simulink model "Sample_Project_s32k144"  (R2019a)
settings: Solver=FixedStepDiscrete  StartTime=0.0  StopTime=10  FixedStep=0.01  RelTol=1e-3
InitFcn:
  | mbd_s32k_consistency_checks(bdroot(gcs));
undefined symbols (not defined in the file): LQFP
libraries: mbd_s32k1xx_ec_toolbox x19, canmsglib x3, simulink x1
Description:
  | This model demonstrate the "GPIO" block functionality.
  | 
  | Validation:
  | - Blue LED is blinking during execution
  | - Press SW2 to light a Green LED
settings Model: Creator=NXP MBDT Team  LastModifiedBy=marsh
settings DataIOCC: ExternalInput=off  InitialState=off  LimitDataPoints=on  SaveFormat=Array  SaveOutput=off  SignalLogging=off  SaveTime=off  ReturnWorkspaceOutputs=off
settings OptimizationCC: DefaultParameterBehavior=Inlined  UseDivisionForNetSlopeComputation=on  GainParamInheritBuiltInType=on  UseFloatMulNetSlope=on  InlineInvariantSignals=on  EnhancedBackFolding=on  PassReuseOutputArgsAs=Individual arguments  ZeroExternalMemoryAtStartup=off  ZeroInternalMemoryAtStartup=off  NoFixptDivByZeroProtection=on  EfficientFloat2IntCast=on  OptimizeBlockOrder=speed  DifferentSizesBufferReuse=on  OptimizationCustomize=off
settings DebuggingCC: UnderspecifiedInitializationDetection=Classic  MergeDetectMultiDrivingBlocksExec=none  SolverPrmCheckMsg=warning  InheritedTsInSrcMsg=none  SingleTaskRateTransMsg=error  ParameterTunabilityLossMsg=error  UnconnectedInputMsg=error  UnconnectedOutputMsg=error  UnconnectedLineMsg=error  AllowSymbolicDim=off  UnknownTsInhSupMsg=error  StateNameClashWarn=warning  SFUnexpectedBacktrackingDiag=warning  SFNoUnconditionalDefaultTransitionDiag=warning  SFExecutionAtInitializationDiag=none  ArithmeticOperatorsInVariantConditions=warning
settings HardwareCC: ProdBitPerPointer=32  ProdBitPerSizeT=32  ProdBitPerPtrDiffT=32  ProdLargestAtomicInteger=Long  ProdLargestAtomicFloat=Double  ProdWordSize=32  ProdLongLongMode=on  ProdHWDeviceType=ARM Compatible->ARM Cortex
settings ModelReferenceCC: PropagateSignalLabelsOutOfModel=off
settings SFSimCC: SimUseLocalCustomCode=off  MATLABDynamicMemAlloc=off
settings RTWCC: SystemTargetFile=mbd_s32k.tlc  MakeCommand=mbd_s32k_make_rtw COPY_MDLREF_INCLUDES=0  TemplateMakefile=mbd_s32k.tmf  Description=Model Based Design Toolbox S32K1xx Code Generation Target  GenerateReport=on  RTWUseLocalCustomCode=off  IncludeHyperlinkInReport=on  LaunchReport=on  GenerateTraceInfo=on  GenerateTraceReport=on  GenerateTraceReportSl=on  GenerateTraceReportSf=on  GenerateTraceReportEml=on  GenerateCodeMetricsReport=on
settings CodeAppCC: ForceParamTrailComments=on  IgnoreCustomStorageClasses=off  OperatorAnnotations=on  SimulinkDataObjDesc=on  SFDataObjDesc=on  CustomSymbolStrGlobalVar=rt$N$M  CustomSymbolStrType=$N$M  CustomSymbolStrFcn=$N$M$F  CustomSymbolStrMacro=$N$M  InsertBlockDesc=on
settings STFCustomTargetCC: TargetLangStandard=C99 (ISO)  MultiwordLength=256  ModelReferenceCompliant=off  CombineOutputUpdateFcns=on  ERTCustomFileBanners=on  SupportContinuousTime=off  SupportNonInlinedSFcns=off  RemoveResetFunc=on  MATLABClassNameForMDSCustomization=Simulink.SoftwareTarget.ERTCustomization  GRTInterface=off  SystemTargetFile=mbd_s32k.tlc
settings ERTTargetCC: TargetLangStandard=C99 (ISO)  ModelReferenceCompliant=off  ParMdlRefBuildCompliant=off  CompOptLevelCompliant=off  ConcurrentExecutionCompliant=off  ModelStepFunctionPrototypeControlCompliant=off  CPPClassGenCompliant=off  UseToolchainInfoCompliant=off  InlinedParameterPlacement=NonHierarchical  ERTCustomFileTemplate=example_file_process.tlc
settings ConfigComp: CovMetricSettings=dw  CovHtmlReporting=on  CovSaveCumulativeToWorkspaceVar=on  CovSaveSingleToWorkspaceVar=on  CovExternalEMLEnable=off

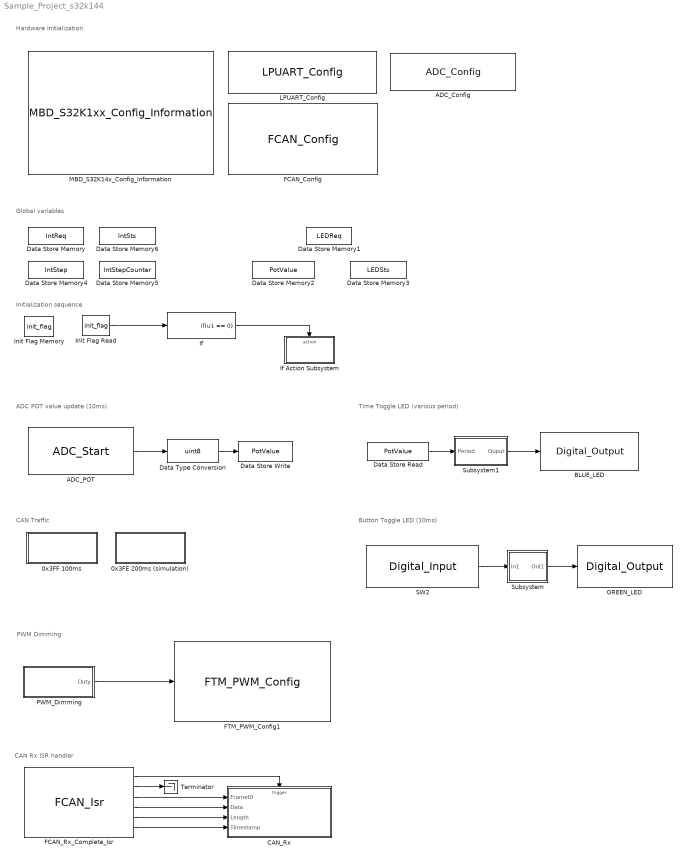
== system Sample_Project_s32k144 ==
  note: ADC POT value update (10ms)
  note: CAN Rx ISR handler
  note: CAN Traffic
  note: Button Toggle LED (10ms)
  note: Time Toggle LED (various period)
  note: Hardware Initialization
  note: Global variables
  note: Initialization sequence
  note: PWM Dimming
  0x3FE 200ms (simulation) : Subsystem
  0x3FF 100ms : Subsystem
  ADC_Config : mbd_s32k1xx_ec_toolbox/Motor Control Blocks/ADC Blocks/ADC_Config  Priority=1  instance=0  mode=8-bit conversion  smplts=29  adiclk=alternate clock 1  adiv=input clock  show_adv_opts=on  pretrgsel=Software pre-trigger  swpretrg=Disabled  adtrg=software  trgsel=PDB output  refsel=Vrefh and Vrefl  supply_monitoring=off  acfe=off  acfgt=off  acren=off  cv1=0  cv2=0  adco=off  avge=off  avgs=4 samples
  ADC_POT : mbd_s32k1xx_ec_toolbox/Motor Control Blocks/ADC Blocks/ADC_Start  Priority=2  instance=0  adc_r=A  adc_chan=PTC14: [ADC0_SE12 | ADC Single Ended Input]  aien=off  mcuTargetUpdate=on
  BLUE_LED : mbd_s32k1xx_ec_toolbox/GPIO Blocks/Digital_Output  gpio_pin=PTD0: [PTD0 | Port D I/O]  init_val=Low  drive_strength=Low
  CAN_Rx : Subsystem  TreatAsAtomicUnit=on
      settings: RTWSystemCode=Nonreusable function
  Data Store Memory : DataStoreMemory  DataStoreName=IntReq  ReadBeforeWriteMsg=warning  WriteAfterWriteMsg=warning  WriteAfterReadMsg=warning  ShowAdditionalParam=off  OutDataTypeStr=uint8
  Data Store Memory1 : DataStoreMemory  DataStoreName=LEDReq  ReadBeforeWriteMsg=warning  WriteAfterWriteMsg=warning  WriteAfterReadMsg=warning  ShowAdditionalParam=off  OutDataTypeStr=boolean
  Data Store Memory2 : DataStoreMemory  DataStoreName=PotValue  ReadBeforeWriteMsg=warning  WriteAfterWriteMsg=warning  WriteAfterReadMsg=warning  InitialValue=0.1  ShowAdditionalParam=off  OutMin=[0.1]  OutMax=[2.65]  OutDataTypeStr=uint8
  Data Store Memory3 : DataStoreMemory  DataStoreName=LEDSts  ReadBeforeWriteMsg=warning  WriteAfterWriteMsg=warning  WriteAfterReadMsg=warning  ShowAdditionalParam=off  OutDataTypeStr=boolean
  Data Store Memory4 : DataStoreMemory  DataStoreName=IntStep  ReadBeforeWriteMsg=warning  WriteAfterWriteMsg=warning  WriteAfterReadMsg=warning  ShowAdditionalParam=off  OutDataTypeStr=double
  Data Store Memory5 : DataStoreMemory  DataStoreName=IntStepCounter  ReadBeforeWriteMsg=warning  WriteAfterWriteMsg=warning  WriteAfterReadMsg=warning  ShowAdditionalParam=off  OutDataTypeStr=uint8
  Data Store Memory6 : DataStoreMemory  DataStoreName=IntSts  ReadBeforeWriteMsg=warning  WriteAfterWriteMsg=warning  WriteAfterReadMsg=warning  ShowAdditionalParam=off  OutDataTypeStr=double
  Data Store Read : DataStoreRead  DataStoreName=PotValue
  Data Store Write : DataStoreWrite  DataStoreName=PotValue
  Data Type Conversion : DataTypeConversion  OutDataTypeStr=uint8
  FCAN_Config : mbd_s32k1xx_ec_toolbox/Communication Blocks/CAN Blocks/FCAN_Config  Priority=1  can_instance=0  can_mode=Loop-back mode  can_max_num_mb=16  can_rx=PTE4: [CAN0_RX | CAN Rx channel]  can_tx=PTE5: [CAN0_TX | CAN Tx Channel]  show_adv_opts=on  can_clk_src=Peripheral clock  bitrate=500  bitrate_adv_opts=off  can_presdiv=7  can_rjw=3  can_pseg1=6  can_pseg2=3  can_propseg=7  can_cbt_presdiv=9  can_cbt_rjw=0  can_cbt_pseg1=3  can_cbt_pseg2=3  can_cbt_propseg=6  can_fd_enable=off  can_payload=8  can_rxfifo_enable=off  can_fifo_id_filter_extended=off  can_fifo_id_filter_remote=off  can_num_id_filters=8  can_fifo_id_format=A  can_fifo_id_filter={'0x0', '0x0', '0x0', '0x0', '0x0', '0x0', '0x0', '0x0'}  can_pn_enable=off  can_wakeup_match=off  can_wakeup_timeout=off  can_timeout_en=off  can_match_timeout=1  can_multiple_matches_en=off  can_num_matches=1  can_idfilter_extendedid=off  can_idfilter_remoteframe=off  can_idfilter_type=Match exact  can_idfilter_id1=0  can_idfilter_id2=0  can_payloadfilter_enable=on  can_payloadfilter_dlclow=0  can_payloadfilter_dlchigh=0  can_payloadfilter_type=Match exact  can_payloadfilter_payload1_b0=0  can_payloadfilter_payload1_b1=0  can_payloadfilter_payload1_b2=0  can_payloadfilter_payload1_b3=0  can_payloadfilter_payload1_b4=0  can_payloadfilter_payload1_b5=0  can_payloadfilter_payload1_b6=0  can_payloadfilter_payload1_b7=0  can_payloadfilter_payload2_b0=0  can_payloadfilter_payload2_b1=0  can_payloadfilter_payload2_b2=0  can_payloadfilter_payload2_b3=0  can_payloadfilter_payload2_b4=0  can_payloadfilter_payload2_b5=0  can_payloadfilter_payload2_b6=0  can_payloadfilter_payload2_b7=0
  FCAN_Rx_Complete_Isr : mbd_s32k1xx_ec_toolbox/Communication Blocks/CAN Blocks/FCAN_Isr  can_instance=0  can_event=Rx Complete
  FTM_PWM_Config1 : mbd_s32k1xx_ec_toolbox/Motor Control Blocks/FTM Blocks/FTM_PWM_Config  Priority=1  ftmModule=0  ftmMode=Edge-Aligned PWM  ftmSourceClock=80 MHz  swcontrol_enable=off  chan0En=on  chan0Type=Complementary  chan2En=off  chan2Type=Independent  chan4En=off  chan4Type=Independent  chan6En=off  chan6Type=Independent  ftmPwmUnits=Hz  outFrequency=5000  ftmPeriod=16000  ftmPrescaler=Divide by 1  deadtimeUnits=Nanoseconds  deadtimeNs=1000  deadtimeTicks=20  deadtimePrescaler=Divide by 4  dutyCycleCh0=0.5  dutyCycleCh1=0.1  dutyCycleCh2=0  dutyCycleCh3=0  dutyCycleCh4=0.25  dutyCycleCh5=0.25  dutyCycleCh6=0.25  dutyCycleCh7=0.25  dutyCycleSim=off  startAfterInit=on  showAdvOpt=on  pinFtmCh0=PTD15: [FTM0_CH0 | FTM Channel]  pinFtmCh1=None  pinPolCh0=Active High  pinPolCh1=Active Low  outputComplem0=Main duplicated  outputLevel0=Low  outputLevel1=Low  pinFtmCh2=PTB14: [FTM0_CH2 | FTM Channel]  pinFtmCh3=None  pinPolCh2=Active High  pinPolCh3=Active Low  outputComplem2=Main duplicated  outputLevel2=Low  outputLevel3=Low  pinFtmCh4=PTB4: [FTM0_CH4 | FTM Channel]  pinFtmCh5=None  pinPolCh4=Active High  pinPolCh5=Active Low  outputComplem4=Main duplicated  outputLevel4=Low  outputLevel5=Low  pinFtmCh6=PTA17: [FTM0_CH6 | FTM Channel]  pinFtmCh7=None  pinPolCh6=Active Low  pinPolCh7=Active Low  outputComplem6=Main duplicated  outputLevel6=Low  outputLevel7=Low  initTrigger=off  chTrigger0=on  chTrigger1=off  chTrigger2=off  chTrigger3=off  chTrigger4=off  chTrigger5=off  chTrigger6=off  chTrigger7=off  mcuTargetUpdate=on  pwmSyncTrg=Software trigger  pwmSyncHwRouting=TRGMUX_FTM7  pwmSyncTrg0=on  pwmSyncTrg1=on  pwmSyncTrg2=on  pwmSyncAutoClear=on  pwmSyncMinLoad=on  pwmSyncMaxLoad=on  pwmSyncInvert=System Clock  pwmSyncOutControl=System Clock  pwmSyncOutMask=System Clock  pwmSyncCounterInitial=System Clock  pwmSyncPoints=Update now  reloadEnable=off  reloadPriority=15  reloadHalfCycle=off  reloadHCR=0  reloadFrequency=0  chnMatch0=off  chnMatch1=off  chnMatch2=off  chnMatch3=off  chnMatch4=off  chnMatch5=off  chnMatch6=off  chnMatch7=off  pwmFaultProtection=off  pwmFaultInterrupt=off  pwmFaultClearing=Automatic Fault control for all channels  pwmFaultPinState=Safe Value  pwmFaultFilterValue=2  pwmFaultPriority=0  fault_disen_0=off  fault_filter_0=off  fault_polarity_0=Active Low  fault_disen_1=off  fault_filter_1=off  fault_polarity_1=Active high  fault_disen_2=off  fault_filter_2=off  fault_polarity_2=Active high  fault_disen_3=off  fault_filter_3=off  fault_polarity_3=Active high  fault_pin_0=None  fault_pin_1=None  fault_pin_2=None  fault_pin_3=None
  GREEN_LED : mbd_s32k1xx_ec_toolbox/GPIO Blocks/Digital_Output  gpio_pin=PTD16: [PTD16 | Port D I/O]  init_val=Low  drive_strength=Low
  If : If  IfExpression=u1 == 0  ShowElse=off
  If Action Subsystem : Subsystem  TreatAsAtomicUnit=on
  Init Flag Memory : DataStoreMemory  DataStoreName=init_flag  ReadBeforeWriteMsg=warning  WriteAfterWriteMsg=warning  WriteAfterReadMsg=warning  ShowAdditionalParam=off  OutDataTypeStr=uint32
  Init Flag Read : DataStoreRead  DataStoreName=init_flag
  LPUART_Config : mbd_s32k1xx_ec_toolbox/Communication Blocks/UART Blocks/LPUART_Config  Priority=1  instance=1  baudrate=115200  databits=8  parity=None  sbns=1  bothedge=rising edge  rxinv=off  txinv=off  show_adv_opts=on  brk13=13 - 16 bit times  lbkde=13 - 16 bit times  rx=PTC6: [LPUART1_RX | Receive]  tx=PTC7: [LPUART1_TX | Transmit]  cts=PTA6: [LPUART1_CTS | Clear To Send (bar)]  rts=PTA7: [LPUART1_RTS | Request To Send]
  MBD_S32K14x_Config_Information : mbd_s32k1xx_ec_toolbox/MBD_S32K1xx_Config_Information  mbdt_ver=0  disp_str=|  config_params=[]  mcu_target_name=S32K144  mcu_target_package=100-LQFP  mcu_target_sram_size=64KB  mcu_system_clock_freq=80  mcu_xtal_freq=External 8  mcu_steptick_timer=LPIT Channel 0  mcu_steptick_prio=15  ds_import_enable=on  target_compiler=GCC  target_memory=FLASH  gcc_target_compile_opts=-mcpu=cortex-m4 -mthumb -mfloat-abi=hard -mfpu=fpv4-sp-d16 -O1 -g -gstrict-dwarf  gcc_target_assemble_opts=-mcpu=cortex-m4 -mthumb -mfloat-abi=hard -mfpu=fpv4-sp-d16 -g  gcc_target_link_opts=-mcpu=cortex-m4 -mthumb -mfloat-abi=hard -mfpu=fpv4-sp-d16  gcc_target_default_lcf=on  gcc_target_user_lcf=S32K148_192_flash.ld  ghs_target_compile_opts=-cpu=cortexm4f -thumb -DARM_MATH_CM4 -fpu=vfpv4_d16 -fsingle -Ogeneral -Wundef -Wimplicit-int -Wshadow -Wtrigraphs --no_commons --gnu_asm -gnu99 -gdwarf-2 -G  ghs_target_assemble_opts=-cpu=cortexm4f -fpu=vfpv4_d16  ghs_target_link_opts=-cpu=cortexm4f -thumb -fpu=vfpv4_d16  ghs_target_default_lcf=on  ghs_target_user_lcf=S32K148_192_flash.ld  iar_target_compile_opts=--cpu=Cortex-M4F --thumb --fpu=VFPv4_sp -Ol -e --debug --dlib_config normal  iar_target_assemble_opts=--cpu Cortex-M4F --thumb --fpu VFPv4_sp  iar_target_link_opts=--no_exceptions --vfe --inline  iar_target_default_lcf=on  iar_target_user_lcf=S32K148_192_flash.icf  pil_download_enable=on  rbl_download_enable=on  rbl_start_delay=5000000  rbl_download_interface=OpenSDA  rbl_restart_request=off  rbl_com_port=COM5  rbl_com_port_custom=COM1  pil_download_rate=115200  pil_opensda_drive=E: EVB-S32K144  pil_opensda_drive_custom=D  pil_uart_instance=1  pil_uart_rx=PTC6: [LPUART1_RX | Receive]  pil_uart_tx=PTC7: [LPUART1_TX | Transmit]  FTM_PWM_PcrCheckEnDis=on  FTM_Input_Edge_Inputs_PcrCheckEnDis=on  FTM_Dual_Edge_Inputs_PcrCheckEnDis=on  FTM_Quadrature_Inputs_PcrCheckEnDis=on  FTM_Hall_Sensor_Inputs_PcrCheckEnDis=on  LPTMR_PcrCheckEnDis=on  PIT_PcrCheckEnDis=on  RTC_PcrCheckEnDis=on  FlexCAN_PcrCheckEnDis=on  LIN_PcrCheckEnDis=on  FlexIO_PcrCheckEnDis=on  LPI2C_PcrCheckEnDis=on  LPSPI_PcrCheckEnDis=on  LPUART_PcrCheckEnDis=on  CMP_PcrCheckEnDis=on  GPIO_OutputPcrCheckEnDis=on  GPIO_InputPcrCheckEnDis=on  SBC_PcrCheckEnDis=on  AMMCLIB_PcrCheckEnDis=on  FM_PcrCheckEnDis=on  Profile_PcrCheckEnDis=on  ConfigParams_PcrCheckEnDis=on  ModelRef_PcrCheckEnDis=on  PDB0_PcrCheckEnDis=on  CSEc_PcrCheckEnDis=on  eDMA_PcrCheckEnDis=on  ADC_PcrCheckEnDis=on  WDOG_PcrCheckEnDis=on
      | Target : S32K144-64KB_SRAM
      | Package : 100-pin
      | System clock : 80 MHz
      | XTAL clock : External 8 MHz
      | Compiler : IAR
      | Target Type : FLASH
      | Download Code after build : off
      | Step Tick Interrupt Priority : 15
  PWM_Dimming : Subsystem
  SW2 : mbd_s32k1xx_ec_toolbox/GPIO Blocks/Digital_Input  gpio_pin=PTC12: [PTC12 | Port C I/O]  pull_resistor=Pulldown  passive_filter=off
  Subsystem : Subsystem
  Subsystem1 : Subsystem
  Terminator : Terminator
  wires:
  SW2/1 -> Subsystem/1(In1)
  Subsystem/1(Out1) -> GREEN_LED/1
  Data Store Read/1 -> Subsystem1/1(Period)
  If/1 -> If Action Subsystem/Action
  Init Flag Read/1 -> If/1
  FCAN_Rx_Complete_Isr/2 -> Terminator/1
  FCAN_Rx_Complete_Isr/4 -> CAN_Rx/2("Data ")
  FCAN_Rx_Complete_Isr/5 -> CAN_Rx/3(Length)
  FCAN_Rx_Complete_Isr/1 -> CAN_Rx/Trigger
  FCAN_Rx_Complete_Isr/3 -> CAN_Rx/1(FrameID)
  FCAN_Rx_Complete_Isr/6 -> CAN_Rx/4(Timestamp)
  ADC_POT/1 -> Data Type Conversion/1
  Data Type Conversion/1 -> Data Store Write/1
  Subsystem1/1(Ouput) -> BLUE_LED/1
  PWM_Dimming/1(Duty) -> FTM_PWM_Config1/1

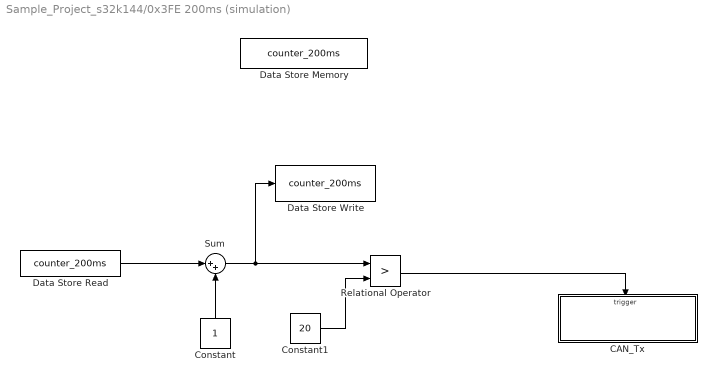
== system Sample_Project_s32k144/0x3FE 200ms (simulation) ==
  CAN_Tx : Subsystem  TreatAsAtomicUnit=on
      settings: RTWSystemCode=Nonreusable function
  Constant : Constant  OutDataTypeStr=uint8
  Constant1 : Constant  Value=20
  Data Store Memory : DataStoreMemory  DataStoreName=counter_200ms  ReadBeforeWriteMsg=warning  WriteAfterWriteMsg=warning  WriteAfterReadMsg=warning  ShowAdditionalParam=off  OutDataTypeStr=uint8
  Data Store Read : DataStoreRead  DataStoreName=counter_200ms
  Data Store Write : DataStoreWrite  DataStoreName=counter_200ms
  Relational Operator : RelationalOperator  Operator=>  OutDataTypeStr=boolean  RndMeth=Simplest
  Sum : Sum  Inputs=|++  AccumDataTypeStr=uint8
  wires:
  Constant1/1 -> Relational Operator/2
  Relational Operator/1 -> CAN_Tx/Trigger
  Constant/1 -> Sum/2
  Sum/1 -> Data Store Write/1, Relational Operator/1
  Data Store Read/1 -> Sum/1

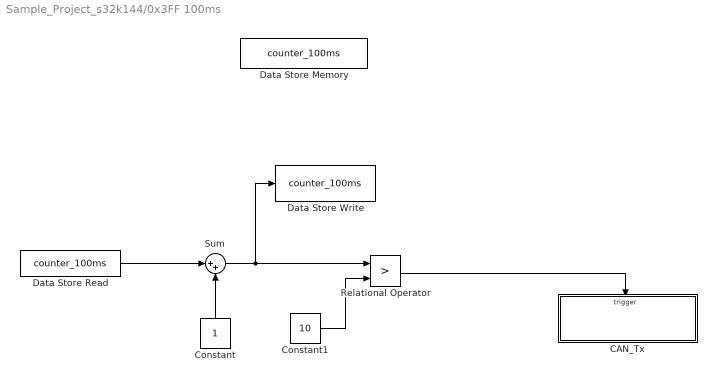
== system Sample_Project_s32k144/0x3FF 100ms ==
  CAN_Tx : Subsystem  TreatAsAtomicUnit=on
      settings: RTWSystemCode=Nonreusable function
  Constant : Constant  OutDataTypeStr=uint8
  Constant1 : Constant  Value=10
  Data Store Memory : DataStoreMemory  DataStoreName=counter_100ms  ReadBeforeWriteMsg=warning  WriteAfterWriteMsg=warning  WriteAfterReadMsg=warning  ShowAdditionalParam=off  OutDataTypeStr=uint8
  Data Store Read : DataStoreRead  DataStoreName=counter_100ms
  Data Store Write : DataStoreWrite  DataStoreName=counter_100ms
  Relational Operator : RelationalOperator  Operator=>  OutDataTypeStr=boolean  RndMeth=Simplest
  Sum : Sum  Inputs=|++  AccumDataTypeStr=uint8
  wires:
  Constant1/1 -> Relational Operator/2
  Relational Operator/1 -> CAN_Tx/Trigger
  Constant/1 -> Sum/2
  Sum/1 -> Data Store Write/1, Relational Operator/1
  Data Store Read/1 -> Sum/1

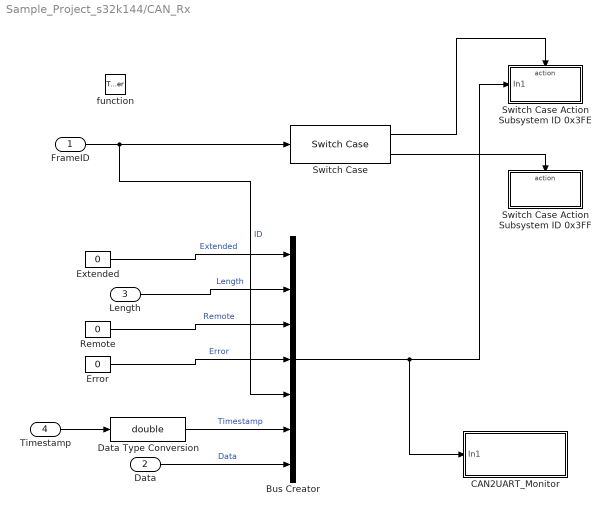
== system Sample_Project_s32k144/CAN_Rx ==
  FrameID : Inport
  "Data " : Inport  Port=2
  Length : Inport  Port=3
  Timestamp : Inport  Port=4
  function : TriggerPort  TriggerType=function-call  VariantControl=Variant
  Bus Creator : BusCreator  Inputs=7  OutDataTypeStr=Bus: CAN_MESSAGE_BUS  NonVirtualBus=on
  CAN2UART_Monitor : Subsystem
  Data Type Conversion : DataTypeConversion  OutDataTypeStr=double
  Error : Constant  Value=0  OutDataTypeStr=uint8
  Extended : Constant  Value=0  OutDataTypeStr=uint8
  Remote : Constant  Value=0  OutDataTypeStr=uint8
  Switch Case : SwitchCase  CaseConditions={hex2dec('3FE'), hex2dec('3FF')}  ShowDefaultCase=off
  Switch Case Action Subsystem ID 0x3FE : Subsystem  TreatAsAtomicUnit=on
  Switch Case Action Subsystem ID 0x3FF : Subsystem  TreatAsAtomicUnit=on
  wires:
  FrameID/1 -> Bus Creator/5, Switch Case/1  "ID"
  Switch Case/1 -> Switch Case Action Subsystem ID 0x3FE/Action
  Switch Case/2 -> Switch Case Action Subsystem ID 0x3FF/Action
  Extended/1 -> Bus Creator/1  "Extended"
  Length/1 -> Bus Creator/2  "Length"
  Remote/1 -> Bus Creator/3  "Remote"
  Error/1 -> Bus Creator/4  "Error"
  "Data "/1 -> Bus Creator/7  "Data"
  Bus Creator/1 -> CAN2UART_Monitor/1(In1), Switch Case Action Subsystem ID 0x3FE/1(In1)
  Data Type Conversion/1 -> Bus Creator/6  "Timestamp"
  Timestamp/1 -> Data Type Conversion/1

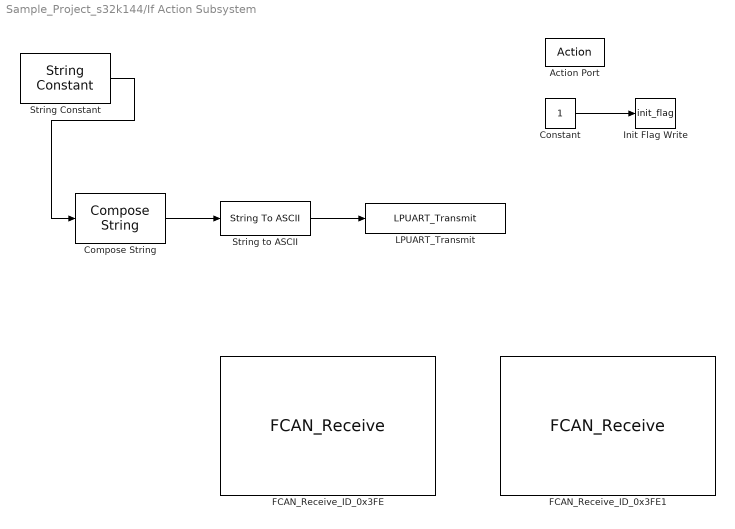
== system Sample_Project_s32k144/If Action Subsystem ==
  Action Port : ActionPort  ActionPortLabel=if(u1 == 0)
  Compose String : ComposeString  Format="\"%s\\n\\r\""
  Constant : Constant  OutDataTypeStr=uint32
  FCAN_Receive_ID_0x3FE : mbd_s32k1xx_ec_toolbox/Communication Blocks/CAN Blocks/FCAN_Receive  can_instance=0  can_mode=Non-blocking  can_timeout_ms=0  can_mb_idx=14  can_extended_id=off  can_is_remote=off  can_id=3FE  can_msg_mask=FFFFFFFF  show_adv_opts=off  can_use_rxfifo=off  can_fd_enable=off
  FCAN_Receive_ID_0x3FE1 : mbd_s32k1xx_ec_toolbox/Communication Blocks/CAN Blocks/FCAN_Receive  can_instance=0  can_mode=Non-blocking  can_timeout_ms=0  can_mb_idx=13  can_extended_id=off  can_is_remote=off  can_id=3FF  can_msg_mask=FFFFFFFF  show_adv_opts=off  can_use_rxfifo=off  can_fd_enable=off
  Init Flag Write : DataStoreWrite  DataStoreName=init_flag
  LPUART_Transmit : mbd_s32k1xx_ec_toolbox/Communication Blocks/UART Blocks/LPUART_Transmit  Priority=2  instance=1
  String Constant : StringConstant  String="\"Start\""
  String to ASCII : StringToASCII  OutputVectorSize=100
  wires:
  Constant/1 -> Init Flag Write/1
  String to ASCII/1 -> LPUART_Transmit/1
  Compose String/1 -> String to ASCII/1
  String Constant/1 -> Compose String/1

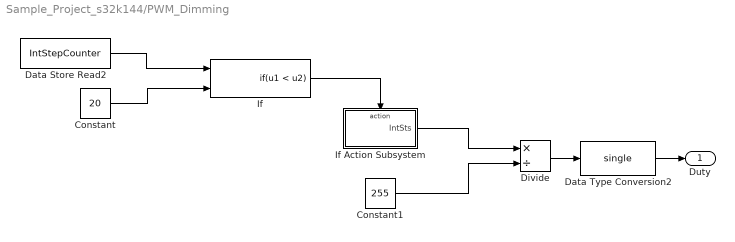
== system Sample_Project_s32k144/PWM_Dimming ==
  Constant : Constant  Value=20  OutDataTypeStr=uint8
  Constant1 : Constant  Value=255
  Data Store Read2 : DataStoreRead  DataStoreName=IntStepCounter
  Data Type Conversion2 : DataTypeConversion  OutDataTypeStr=single
  Divide : Product  Inputs=*/
  If : If  NumInputs=2  IfExpression=u1 < u2  ShowElse=off
  If Action Subsystem : Subsystem  TreatAsAtomicUnit=on
  Duty : Outport
  wires:
  Data Store Read2/1 -> If/1
  Constant/1 -> If/2
  If/1 -> If Action Subsystem/Action
  If Action Subsystem/1(IntSts) -> Divide/1
  Constant1/1 -> Divide/2
  Data Type Conversion2/1 -> Duty/1
  Divide/1 -> Data Type Conversion2/1

== system Sample_Project_s32k144/Subsystem ==
  In1 : Inport
  Chart : Stateflow chart  BlockKeywords=__PRM__SERIALIZED__DATA__:Stateflow Chart,Stateflow Diagram  TreatAsAtomicUnit=on
  Scope1 : Scope  NumInputPorts=3
  Subsystem : Subsystem
  Out1 : Outport
  wires:
  In1/1 -> Scope1/1, Chart/1(sw)
  Chart/1(y) -> Subsystem/Trigger, Scope1/2
  Subsystem/1(Out1) -> Out1/1, Scope1/3

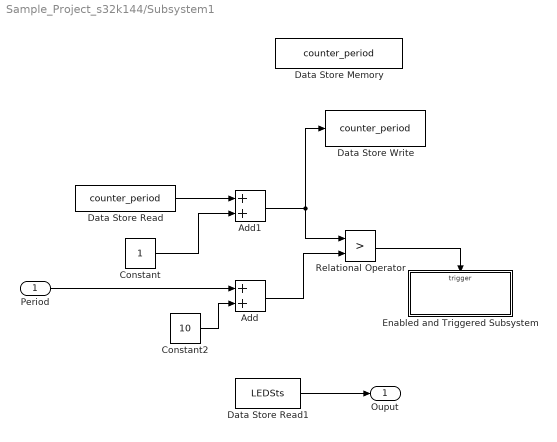
== system Sample_Project_s32k144/Subsystem1 ==
  Period : Inport
  Add : Sum
  Add1 : Sum
  Constant : Constant  OutDataTypeStr=uint8
  Constant2 : Constant  Value=10
  Data Store Memory : DataStoreMemory  DataStoreName=counter_period  ReadBeforeWriteMsg=warning  WriteAfterWriteMsg=warning  WriteAfterReadMsg=warning  ShowAdditionalParam=off  OutDataTypeStr=uint32
  Data Store Read : DataStoreRead  DataStoreName=counter_period
  Data Store Read1 : DataStoreRead  DataStoreName=LEDSts
  Data Store Write : DataStoreWrite  DataStoreName=counter_period
  Enabled and Triggered Subsystem : Subsystem  TreatAsAtomicUnit=on
  Relational Operator : RelationalOperator  Operator=>  OutDataTypeStr=boolean  RndMeth=Simplest
  Ouput : Outport
  wires:
  Data Store Read1/1 -> Ouput/1
  Data Store Read/1 -> Add1/1
  Constant/1 -> Add1/2
  Constant2/1 -> Add/2
  Add1/1 -> Data Store Write/1, Relational Operator/1
  Add/1 -> Relational Operator/2
  Relational Operator/1 -> Enabled and Triggered Subsystem/Trigger
  Period/1 -> Add/1

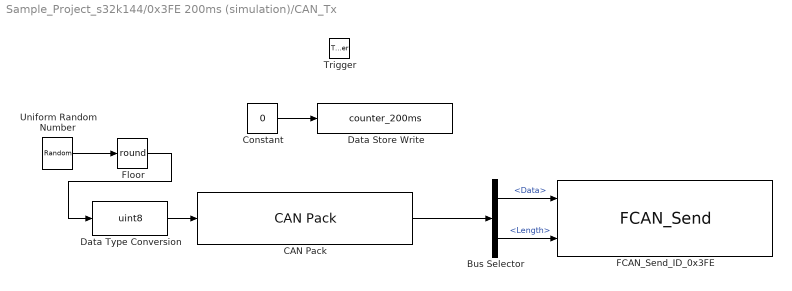
== system Sample_Project_s32k144/0x3FE 200ms (simulation)/CAN_Tx ==
  Trigger : TriggerPort  VariantControl=Variant  PortDimensions=1
  Bus Selector : BusSelector  OutputSignals=Data,Length
  CAN Pack : canmsglib/CAN Pack  CANdbFile=D:\AUTOSAR\Project\Simulink_Project\dbc\CAN1.dbc  MsgList=ECU1_01_3FE  MsgName=ECU1_01_3FE  MsgIDType=Standard (11-bit identifier)  MsgIdentifier=1022  MsgLength=8  SignalInfo=IntReq$0$8$2$2$1$0$1$0$0$255$#  NSignals=1  StartBits=str2num('[int32(0)]')  SignalSizes=str2num('[int32(8)]')  ByteOrders=str2num('[int32(2)]')  DataTypes=str2num('[int32(2)]')  MultiplexTypes=str2num('[int32(1)]')  MultiplexValues=str2num('[double(0)]')  Factors=str2num('[double(1)]')  Offsets=str2num('[double(0)]')  Minimums=str2num('[double(0)]')  Maximums=str2num('[double(255)]')  Remote=off  ApplyMinMax=off  BusOutput=on
      settings: SourceProductName=Vehicle Network Toolbox  SourceProductBaseCode=VN  DataFormat=CANdb specified signals
  Constant : Constant  Value=0  OutDataTypeStr=uint8
  Data Store Write : DataStoreWrite  DataStoreName=counter_200ms
  Data Type Conversion : DataTypeConversion  OutDataTypeStr=uint8
  FCAN_Send_ID_0x3FE : mbd_s32k1xx_ec_toolbox/Communication Blocks/CAN Blocks/FCAN_Send  Priority=2  can_instance=0  can_mode=Non-blocking  can_timeout_ms=0  can_mb_idx=1  can_extended_id=off  can_is_remote=off  can_id=3FE  show_adv_opts=on  can_fd_enable=off  can_enable_brs=off  can_fd_padding=0
  Floor : Rounding  Operator=round
  Uniform Random Number : UniformRandomNumber  Minimum=0  Maximum=255  Seed=21
  wires:
  Constant/1 -> Data Store Write/1
  CAN Pack/1 -> Bus Selector/1
  Bus Selector/1 -> FCAN_Send_ID_0x3FE/1  "<Data>"
  Bus Selector/2 -> FCAN_Send_ID_0x3FE/2  "<Length>"
  Data Type Conversion/1 -> CAN Pack/1
  Uniform Random Number/1 -> Floor/1
  Floor/1 -> Data Type Conversion/1

== system Sample_Project_s32k144/0x3FF 100ms/CAN_Tx ==
  Trigger : TriggerPort  VariantControl=Variant  PortDimensions=1
  Bus Selector : BusSelector  OutputSignals=Data,Length
  CAN Pack : canmsglib/CAN Pack  CANdbFile=D:\AUTOSAR\Project\Simulink_Project\dbc\CAN1.dbc  MsgList=ECU2_01_3FF  MsgName=ECU2_01_3FF  MsgIDType=Standard (11-bit identifier)  MsgIdentifier=1023  MsgLength=8  SignalInfo=LEDSts$39$1$2$2$1$0$1$0$0$1$#PotValue$0$8$2$2$1$0$1$0$0$255$#  NSignals=2  StartBits=str2num('[int32(39);int32(0)]')  SignalSizes=str2num('[int32(1);int32(8)]')  ByteOrders=str2num('[int32(2);int32(2)]')  DataTypes=str2num('[int32(2);int32(2)]')  MultiplexTypes=str2num('[int32(1);int32(1)]')  MultiplexValues=str2num('[double(0);double(0)]')  Factors=str2num('[double(1);double(1)]')  Offsets=str2num('[double(0);double(0)]')  Minimums=str2num('[double(0);double(0)]')  Maximums=str2num('[double(1);double(255)]')  Remote=off  ApplyMinMax=off  BusOutput=on
      settings: SourceProductName=Vehicle Network Toolbox  SourceProductBaseCode=VN  DataFormat=CANdb specified signals
  Constant : Constant  Value=0  OutDataTypeStr=uint8
  Data Store Read : DataStoreRead  DataStoreName=PotValue
  Data Store Read1 : DataStoreRead  DataStoreName=LEDSts
  Data Store Write : DataStoreWrite  DataStoreName=counter_100ms
  FCAN_Send_ID_0x3FF : mbd_s32k1xx_ec_toolbox/Communication Blocks/CAN Blocks/FCAN_Send  Priority=2  can_instance=0  can_mode=Non-blocking  can_timeout_ms=0  can_mb_idx=0  can_extended_id=off  can_is_remote=off  can_id=3FF  show_adv_opts=on  can_fd_enable=off  can_enable_brs=off  can_fd_padding=0
  wires:
  Data Store Read1/1 -> CAN Pack/1
  Data Store Read/1 -> CAN Pack/2
  Constant/1 -> Data Store Write/1
  CAN Pack/1 -> Bus Selector/1
  Bus Selector/1 -> FCAN_Send_ID_0x3FF/1  "<Data>"
  Bus Selector/2 -> FCAN_Send_ID_0x3FF/2  "<Length>"

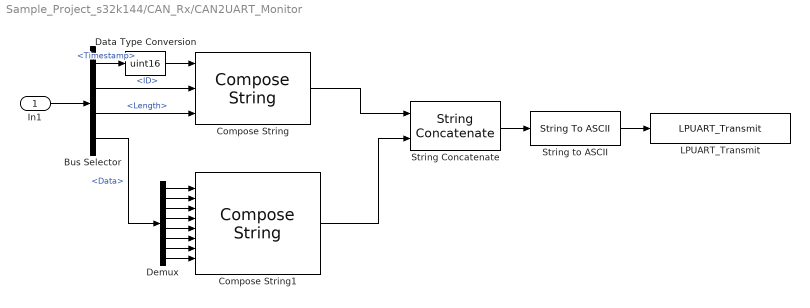
== system Sample_Project_s32k144/CAN_Rx/CAN2UART_Monitor ==
  In1 : Inport  OutDataTypeStr=Bus: CAN_MESSAGE_BUS
  Bus Selector : BusSelector  OutputSignals=Timestamp,ID,Length,Data
  Compose String : ComposeString  Format="\"%u\\t0x%X\\t%u\\t\""
  Compose String1 : ComposeString  Format="\"%.2X %.2X %.2X %.2X %.2X %.2X %.2X %.2X \\r\\n\""
  Data Type Conversion : DataTypeConversion  OutDataTypeStr=uint16
  Demux : Demux  Outputs=8
  LPUART_Transmit : mbd_s32k1xx_ec_toolbox/Communication Blocks/UART Blocks/LPUART_Transmit  Priority=2  instance=1
  String Concatenate : StringConcatenate
  String to ASCII : StringToASCII  OutputVectorSize=100
  wires:
  String to ASCII/1 -> LPUART_Transmit/1
  Compose String/1 -> String Concatenate/1
  In1/1 -> Bus Selector/1
  Bus Selector/2 -> Compose String/2  "<ID>"
  Bus Selector/3 -> Compose String/3  "<Length>"
  Data Type Conversion/1 -> Compose String/1
  Bus Selector/1 -> Data Type Conversion/1  "<Timestamp>"
  Compose String1/1 -> String Concatenate/2
  String Concatenate/1 -> String to ASCII/1
  Bus Selector/4 -> Demux/1  "<Data>"
  Demux/1 -> Compose String1/1
  Demux/2 -> Compose String1/2
  Demux/3 -> Compose String1/3
  Demux/4 -> Compose String1/4
  Demux/5 -> Compose String1/5
  Demux/6 -> Compose String1/6
  Demux/7 -> Compose String1/7
  Demux/8 -> Compose String1/8

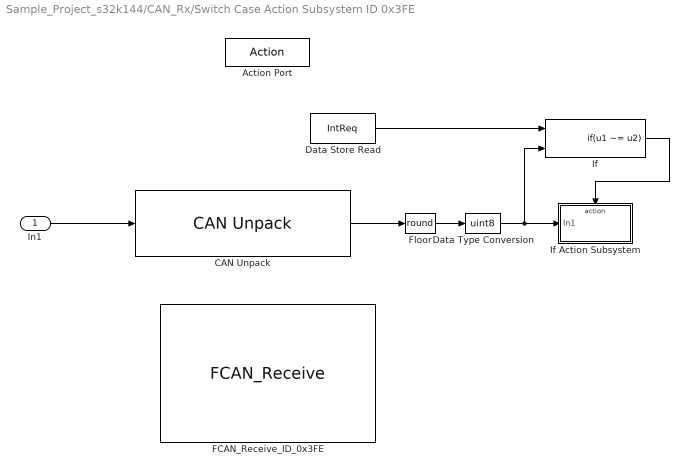
== system Sample_Project_s32k144/CAN_Rx/Switch Case Action Subsystem ID 0x3FE ==
  In1 : Inport  OutDataTypeStr=Bus: CAN_MESSAGE_BUS
  Action Port : ActionPort  ActionPortLabel=case [ 1022 ]:
  CAN Unpack : canmsglib/CAN Unpack  CANdbFile=D:\AUTOSAR\Project\Simulink_Project\dbc\CAN1.dbc  MsgList=ECU1_01_3FE  MsgName=ECU1_01_3FE  MsgIDType=Standard (11-bit identifier)  MsgIdentifier=1022  MsgLength=8  SignalInfo=IntReq$0$8$2$2$1$0$1$0$0$255$#  NSignals=1  IDPort=off  TimestampPort=off  ErrorPort=off  RemotePort=off  LengthPort=off  StatusPort=off  StartBits=str2num('[int32(0)]')  SignalSizes=str2num('[int32(8)]')  ByteOrders=str2num('[int32(2)]')  DataTypes=str2num('[int32(2)]')  MultiplexTypes=str2num('[int32(1)]')  MultiplexValues=str2num('[double(0)]')  Factors=str2num('[double(1)]')  Offsets=str2num('[double(0)]')  Minimums=str2num('[double(0)]')  Maximums=str2num('[double(255)]')  ApplyMinMax=off
      settings: SourceProductName=Vehicle Network Toolbox  SourceProductBaseCode=VN  DataFormat=CANdb specified signals
  Data Store Read : DataStoreRead  DataStoreName=IntReq
  Data Type Conversion : DataTypeConversion  OutDataTypeStr=uint8
  FCAN_Receive_ID_0x3FE : mbd_s32k1xx_ec_toolbox/Communication Blocks/CAN Blocks/FCAN_Receive  can_instance=0  can_mode=Non-blocking  can_timeout_ms=0  can_mb_idx=14  can_extended_id=off  can_is_remote=off  can_id=3FE  can_msg_mask=FFFFFFFF  show_adv_opts=off  can_use_rxfifo=off  can_fd_enable=off
  Floor : Rounding  Operator=round
  If : If  NumInputs=2  IfExpression=u1 ~= u2  ShowElse=off
  If Action Subsystem : Subsystem  TreatAsAtomicUnit=on
  wires:
  In1/1 -> CAN Unpack/1
  If/1 -> If Action Subsystem/Action
  Data Store Read/1 -> If/1
  Data Type Conversion/1 -> If/2, If Action Subsystem/1(In1)
  Floor/1 -> Data Type Conversion/1
  CAN Unpack/1 -> Floor/1

== system Sample_Project_s32k144/CAN_Rx/Switch Case Action Subsystem ID 0x3FF ==
  Action Port : ActionPort  ActionPortLabel=case [ 1023 ]:
  FCAN_Receive_ID_0x3FF : mbd_s32k1xx_ec_toolbox/Communication Blocks/CAN Blocks/FCAN_Receive  can_instance=0  can_mode=Non-blocking  can_timeout_ms=0  can_mb_idx=13  can_extended_id=off  can_is_remote=off  can_id=3FF  can_msg_mask=FFFFFFFF  show_adv_opts=off  can_use_rxfifo=off  can_fd_enable=off

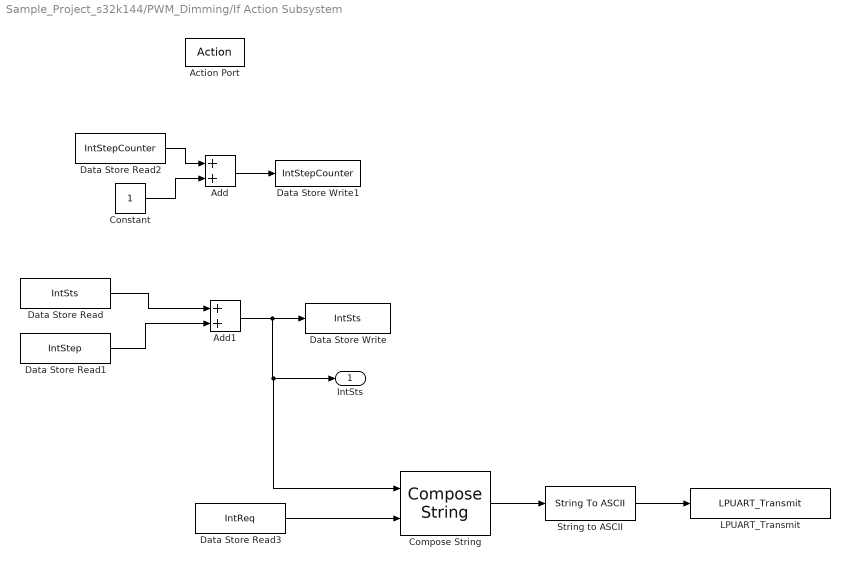
== system Sample_Project_s32k144/PWM_Dimming/If Action Subsystem ==
  Action Port : ActionPort  ActionPortLabel=if(u1 < u2)
  Add : Sum
  Add1 : Sum
  Compose String : ComposeString  Format="\"IntSts:%3.3f\\tIntReq:%u\\n\\r\""
  Constant : Constant  OutDataTypeStr=uint8
  Data Store Read : DataStoreRead  DataStoreName=IntSts
  Data Store Read1 : DataStoreRead  DataStoreName=IntStep
  Data Store Read2 : DataStoreRead  DataStoreName=IntStepCounter
  Data Store Read3 : DataStoreRead  DataStoreName=IntReq
  Data Store Write : DataStoreWrite  DataStoreName=IntSts
  Data Store Write1 : DataStoreWrite  DataStoreName=IntStepCounter
  LPUART_Transmit : mbd_s32k1xx_ec_toolbox/Communication Blocks/UART Blocks/LPUART_Transmit  Priority=2  instance=1
  String to ASCII : StringToASCII  OutputVectorSize=100
  IntSts : Outport
  wires:
  Constant/1 -> Add/2
  Add/1 -> Data Store Write1/1
  Data Store Read1/1 -> Add1/2
  Add1/1 -> Compose String/1, IntSts/1, Data Store Write/1
  Data Store Read2/1 -> Add/1
  Data Store Read/1 -> Add1/1
  String to ASCII/1 -> LPUART_Transmit/1
  Compose String/1 -> String to ASCII/1
  Data Store Read3/1 -> Compose String/2

== system Sample_Project_s32k144/Subsystem/Subsystem ==
  Trigger : TriggerPort  VariantControl=Variant  PortDimensions=1
  Bitwise Operator : simulink/Logic and Bit Operations/Bitwise Operator  logicop=NOT  UseBitMask=off  BitMask=bin2dec('11011001')  BitMaskRealWorld=Stored Integer
  Data Store Memory : DataStoreMemory  DataStoreName=LedSts  ReadBeforeWriteMsg=warning  WriteAfterWriteMsg=warning  WriteAfterReadMsg=warning  ShowAdditionalParam=off  OutDataTypeStr=boolean
  Data Store Read : DataStoreRead  DataStoreName=LedSts
  Data Store Write : DataStoreWrite  DataStoreName=LedSts
  Out1 : Outport
  wires:
  Data Store Read/1 -> Bitwise Operator/1
  Bitwise Operator/1 -> Data Store Write/1, Out1/1

== system Sample_Project_s32k144/Subsystem1/Enabled and Triggered Subsystem ==
  Trigger : TriggerPort  VariantControl=Variant
  Constant : Constant  Value=0  OutDataTypeStr=Inherit: Inherit via back propagation
  Data Store Read1 : DataStoreRead  DataStoreName=LEDSts
  Data Store Write : DataStoreWrite  DataStoreName=counter_period
  Data Store Write1 : DataStoreWrite  DataStoreName=LEDSts
  Logical Operator : Logic  Operator=NOT  AllPortsSameDT=off  OutDataTypeStr=boolean
  wires:
  Data Store Read1/1 -> Logical Operator/1
  Logical Operator/1 -> Data Store Write1/1
  Constant/1 -> Data Store Write/1

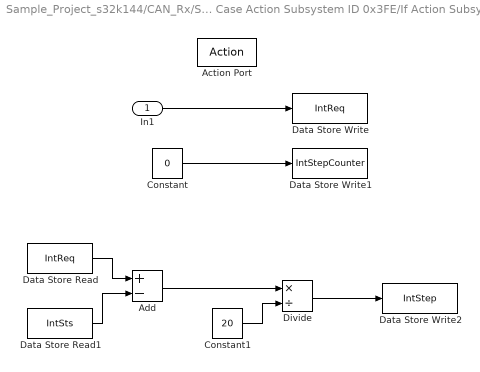
== system Sample_Project_s32k144/CAN_Rx/Switch Case Action Subsystem ID 0x3FE/If Action Subsystem ==
  In1 : Inport
  Action Port : ActionPort  ActionPortLabel=if(u1 ~= u2)
  Add : Sum  Inputs=+-
  Constant : Constant  Value=0  OutDataTypeStr=uint8
  Constant1 : Constant  Value=20
  Data Store Read : DataStoreRead  DataStoreName=IntReq
  Data Store Read1 : DataStoreRead  DataStoreName=IntSts
  Data Store Write : DataStoreWrite  DataStoreName=IntReq
  Data Store Write1 : DataStoreWrite  DataStoreName=IntStepCounter
  Data Store Write2 : DataStoreWrite  DataStoreName=IntStep
  Divide : Product  Inputs=*/
  wires:
  In1/1 -> Data Store Write/1
  Constant/1 -> Data Store Write1/1
  Data Store Read/1 -> Add/1
  Data Store Read1/1 -> Add/2
  Add/1 -> Divide/1
  Constant1/1 -> Divide/2
  Divide/1 -> Data Store Write2/1

== stateflow chart Sample_Project_s32k144/Subsystem/Chart ==
  state BtnNotPressed
    y = 0;
  state BtnPressed
    y = 1;
  (default) -> BtnNotPressed
  BtnPressed -> BtnNotPressed : [duration(sw==0) < 0.01]
  BtnNotPressed -> BtnPressed : [duration(sw>0) > 0.1]
  data: sw input; y output
